simulink model "model"  (Simulink 7.3)
settings: Solver=ode45  StartTime=0.0  StopTime=10.0  RelTol=1e-3
values from neighbouring files (symbols this model uses):
  K = 0    [az.m]    (also in az_.m = 324.324324324; az_2.m = 324.324324324; az_3.m = 324.324324324; az_d.m = 700)
undefined symbols (not defined in the file or in its folder): alpha, Kd, Kdus, tau, Tdus
settings Model: Creator=Sainquake  LastModifiedBy=Sainquake

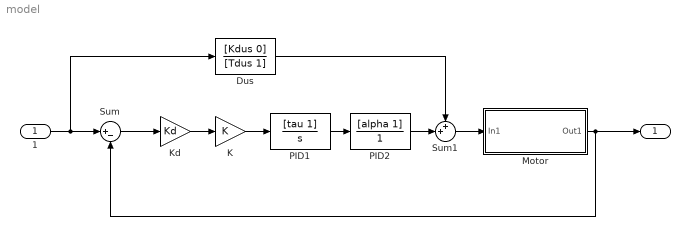
== system model ==
  " 1" : Inport  OutDataType=fixdt(1, 16)  OutScaling=2^0
  " Kd" : Gain  Gain=Kd  ParameterDataType=fixdt(1, 16)  ParameterScaling=2^0  OutDataType=fixdt(1, 16)  OutScaling=2^0
  Dus : TransferFcn  Numerator=[Kdus 0]  Denominator=[Tdus 1]
  K : Gain  Gain=K  ParameterDataType=fixdt(1, 16)  ParameterScaling=2^0  OutDataType=fixdt(1, 16)  OutScaling=2^0
  Motor : Subsystem
  PID1 : TransferFcn  Numerator=[tau 1]  Denominator=[1 0]
  PID2 : TransferFcn  Numerator=[alpha 1]  Denominator=[1]
  Sum : Sum  Inputs=|+-  OutDataType=fixdt(1, 16)  OutScaling=2^0
  Sum1 : Sum  Inputs=++|  OutDataType=fixdt(1, 16)  OutScaling=2^0
  " " : Outport  OutDataType=fixdt(1, 16)  OutScaling=2^0
  wires:
  PID2/1 -> Sum1/2
  PID1/1 -> PID2/1
  K/1 -> PID1/1
  " Kd"/1 -> K/1
  Sum/1 -> " Kd"/1
  Dus/1 -> Sum1/1
  Sum1/1 -> Motor/1(In1)
  Motor/1(Out1) -> " "/1, Sum/2
  " 1"/1 -> Sum/1, Dus/1

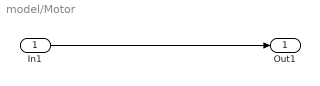
== system model/Motor ==
  In1 : Inport  OutDataType=fixdt(1, 16)  OutScaling=2^0
  Out1 : Outport  OutDataType=fixdt(1, 16)  OutScaling=2^0
  wires:
  In1/1 -> Out1/1
